simulink model "sm_controlled_current_boost"  (R2016a)
settings: Solver=VariableStepAuto  StartTime=0.0  StopTime=5  RelTol=1e-3
libraries: powerlib x11
settings Model: Creator=jorda  LastModifiedBy=jorda

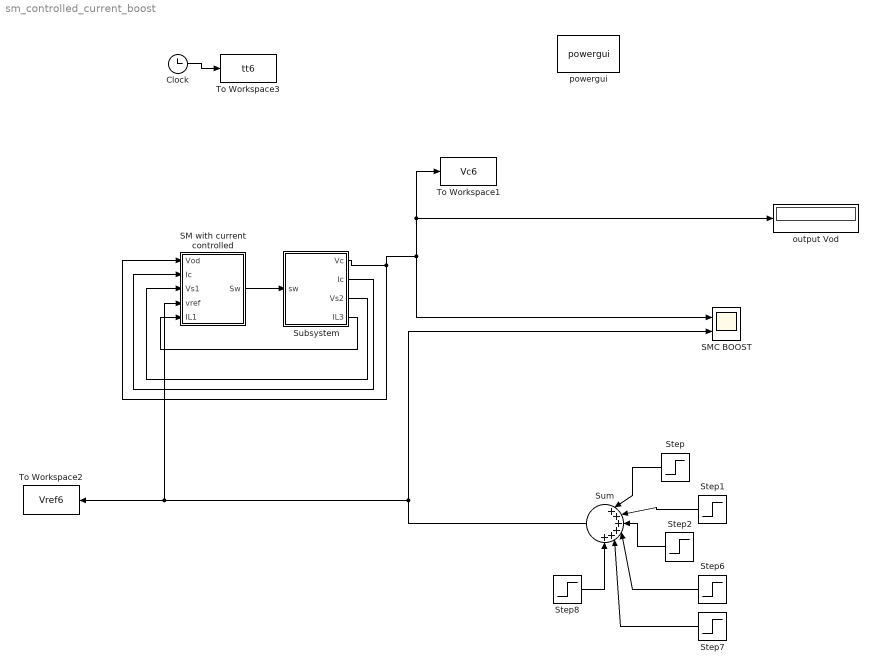
== system sm_controlled_current_boost ==
  Clock : Clock
  SM with current controlled : Subsystem
  SMC BOOST : Scope  NumInputPorts=2
  Step : Step  Time=0.5  Before=20  After=21  SampleTime=0
  Step1 : Step  SampleTime=0
  Step2 : Step  Time=1.5  After=-2  SampleTime=0
  Step6 : Step  Time=2  After=-1  SampleTime=0
  Step7 : Step  Time=2.5  After=-1  SampleTime=0
  Step8 : Step  Time=3  After=2  SampleTime=0
  Subsystem : Subsystem
  Sum : Sum  Inputs=|++++++
  To Workspace1 : ToWorkspace  VariableName=Vc6  SampleTime=1e-3
  To Workspace2 : ToWorkspace  VariableName=Vref6  SampleTime=1e-3
  To Workspace3 : ToWorkspace  VariableName=tt6  SampleTime=1e-3
  output Vod : Display
  powergui : powerlib/powergui  Priority=1  SimulationMode=Continuous  SolverType=Tustin/Backward Euler (TBE)  SampleTime=50e-6  frequency=60  SPID=off  DisableSnubberDevices=off  DisableRonSwitches=off  DisableVfSwitches=off  SwTol=0  DisplayEquations=off  Interpol=off  ExternalGateDelay=off  methode=off  Ts=10  FunctionMessages=off  echomessages=off  HookPort=off  EnableUseOfTLC=off  x0status=blocks  frequencyindice=0  Pbase=100e6  ErrMax=1e-4  Iterations=50  UnitsV=kV  UnitsW=MW  buscounter=0  RestoreLinks=warning  ResistiveCurrentMeasurement=off  Frange=[0:2:500]  Ylog=off  Xlog=on  ShowGrid=off  save=off  variable=ZData  structure=0  ZoomFFT=off  StartTime=0.0  cycles=1  DisplayStyle=1  fundamental=60  FreqAxis=off  MaxFrequency=1000  frequencyindicesteady=1  RmsSteady=1  display=off
  wires:
  SM with current controlled/1(Sw) -> Subsystem/1(sw)
  Sum/1 -> To Workspace2/1, SM with current controlled/4(vref), SMC BOOST/2
  Subsystem/1(Vc) -> To Workspace1/1, output Vod/1, SMC BOOST/1, SM with current controlled/1(Vod)
  Subsystem/2(Ic) -> SM with current controlled/2(Ic)
  Subsystem/3(Vs2) -> SM with current controlled/3("Vs1 ")
  Step/1 -> Sum/1
  Step1/1 -> Sum/2
  Step2/1 -> Sum/3
  Step6/1 -> Sum/4
  Step7/1 -> Sum/5
  Step8/1 -> Sum/6
  Subsystem/4(IL3) -> SM with current controlled/5(IL1)
  Clock/1 -> To Workspace3/1

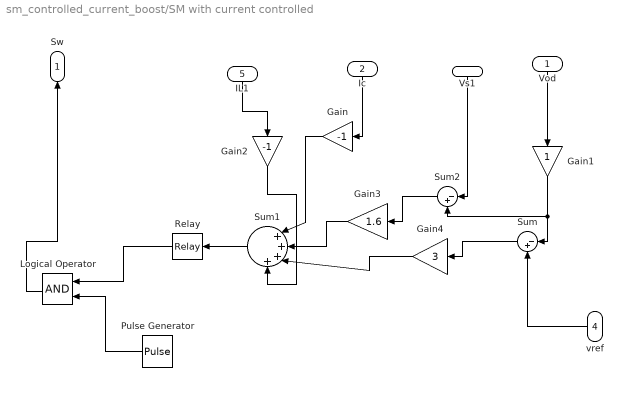
== system sm_controlled_current_boost/SM with current controlled ==
  Vod : Inport
  Ic : Inport  Port=2
  "Vs1 " : Inport  Port=3
  vref : Inport  Port=4
  IL1 : Inport  Port=5
  Gain : Gain  Gain=-1  ParamDataTypeStr=double  OutDataTypeStr=double
  Gain1 : Gain  ParamDataTypeStr=double  OutDataTypeStr=double
  Gain2 : Gain  Gain=-1  ParamDataTypeStr=double  OutDataTypeStr=double
  Gain3 : Gain  Gain=1.6  ParamDataTypeStr=double  OutDataTypeStr=double
  Gain4 : Gain  Gain=3  ParamDataTypeStr=double  OutDataTypeStr=double
  Logical Operator : Logic  AllPortsSameDT=off  OutDataTypeStr=boolean
  Pulse Generator : DiscretePulseGenerator  PulseType=Time based  Period=1e-3  PulseWidth=50
  Relay : Relay  OnSwitchValue=0.2  OffSwitchValue=-0.2  OutDataTypeStr=Inherit: Inherit via back propagation
  Sum : Sum  Inputs=|-+  AccumDataTypeStr=single  OutDataTypeStr=double  InputSameDT=on
  Sum1 : Sum  Inputs=|++++  AccumDataTypeStr=double  OutDataTypeStr=double  InputSameDT=on
  Sum2 : Sum  Inputs=|-+  AccumDataTypeStr=single  OutDataTypeStr=double  InputSameDT=on
  Sw : Outport
  wires:
  Gain1/1 -> Sum2/2, Sum/1
  "Vs1 "/1 -> Sum2/1
  Vod/1 -> Gain1/1
  Ic/1 -> Gain/1
  vref/1 -> Sum/2
  Sum/1 -> Gain4/1
  Sum2/1 -> Gain3/1
  Gain/1 -> Sum1/1
  Gain3/1 -> Sum1/2
  Gain4/1 -> Sum1/3
  Relay/1 -> Logical Operator/1
  Pulse Generator/1 -> Logical Operator/2
  Logical Operator/1 -> Sw/1
  Sum1/1 -> Relay/1
  IL1/1 -> Gain2/1
  Gain2/1 -> Sum1/4

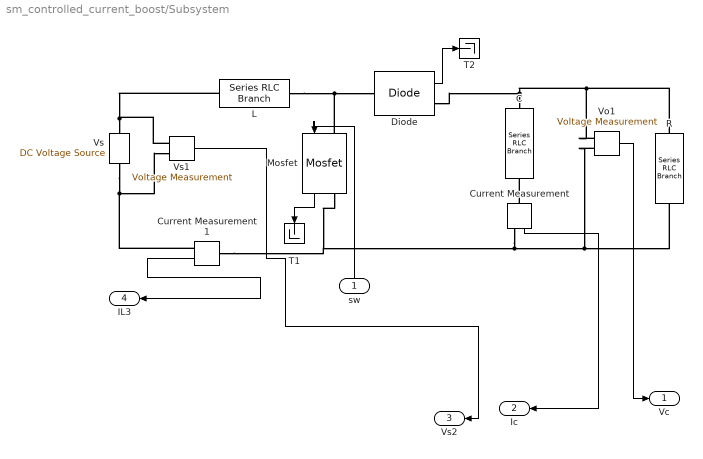
== system sm_controlled_current_boost/Subsystem ==
  sw : Inport
  C : powerlib/Elements/Series RLC Branch  LConnTagsString=__new0  RConnTagsString=__new0  BranchType=C  Resistance=1  Inductance=1e-3  SetiL0=off  InitialCurrent=0  Capacitance=2000e-6  Setx0=off  InitialVoltage=0  Measurements=None
  Current Measurement : powerlib/Measurements/Current Measurement  PhasorSimulation=off  OutputType=Complex  PSBequivalent=0
  Current Measurement1 : powerlib/Measurements/Current Measurement  PhasorSimulation=off  OutputType=Complex  PSBequivalent=0
  Diode : powerlib/Power Electronics/Diode  Ron=0.001  Lon=0  Vf=0.8  IC=0  UseSnubber=off  Rs=500  Cs=250e-9  Measurements=on
  L : powerlib/Elements/Series RLC Branch  LConnTagsString=__new0  RConnTagsString=__new0  BranchType=L  Resistance=1  Inductance=2e-3  SetiL0=off  InitialCurrent=0  Capacitance=1e-6  Setx0=off  InitialVoltage=0  Measurements=None
  Mosfet : powerlib/Power Electronics/Mosfet  Ron=0.1  Lon=0  Rd=0.01  Vfd=0  IC=0  Rs=1e5  Cs=inf  Measurements=on
  R : powerlib/Elements/Series RLC Branch  LConnTagsString=__new0  RConnTagsString=__new0  BranchType=R  Resistance=4  Inductance=1e-3  SetiL0=off  InitialCurrent=0  Capacitance=1e-6  Setx0=off  InitialVoltage=0  Measurements=None
  T1 : Terminator
  T2 : Terminator
  Vo1 : powerlib/Measurements/Voltage Measurement  PhasorSimulation=off  OutputType=Complex  PSBequivalent=0
  Vs : powerlib/Electrical Sources/DC Voltage Source  Amplitude=15  Measurements=None
  Vs1 : powerlib/Measurements/Voltage Measurement  PhasorSimulation=off  OutputType=Complex  PSBequivalent=0
  Vc : Outport
  Ic : Outport  Port=2
  Vs2 : Outport  Port=3
  IL3 : Outport  Port=4
  wires:
  Vs1/1 -> Vs2/1
  Mosfet/1 -> T1/1
  Current Measurement/1 -> Ic/1
  Vo1/1 -> Vc/1
  Diode/1 -> T2/1
  sw/1 -> Mosfet/1
  Current Measurement1/1 -> IL3/1
  connections:
  Vs/RConn1 -- L/LConn1 -- Vs1/LConn1
  Current Measurement/RConn1 -- Mosfet/RConn1 -- Current Measurement1/LConn1 -- Vo1/LConn2 -- R/RConn1
  L/RConn1 -- Mosfet/LConn1 -- Diode/LConn1
  R/LConn1 -- Vo1/LConn1 -- Diode/RConn1 -- C/LConn1
  Current Measurement/LConn1 -- C/RConn1
  Vs/LConn1 -- Current Measurement1/RConn1 -- Vs1/LConn2
